simulink model "HPFilter"  (R2020b)
settings: Solver=VariableStepAuto  StartTime=0.0  StopTime=0.1  RelTol=1e-3
settings Model: Creator=Admin  LastModifiedBy=Admin

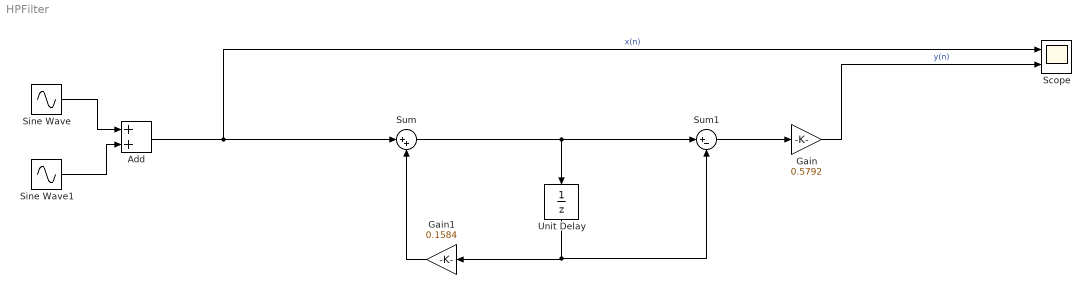
== system HPFilter ==
  Add : Sum
  Gain : Gain  Gain=0.5792
  Gain1 : Gain  Gain=0.1584
  Scope : Scope  NumInputPorts=2
  Sine Wave : Sin  Frequency=200/2*pi  SampleTime=0
  Sine Wave1 : Sin  Amplitude=0.25  Frequency=1000/2*pi  SampleTime=0
  Sum : Sum  Inputs=|++
  Sum1 : Sum  Inputs=|+-
  Unit Delay : UnitDelay  SampleTime=-1  HasFrameUpgradeWarning=on
  wires:
  Sum/1 -> Unit Delay/1, Sum1/1
  Sine Wave/1 -> Add/1
  Unit Delay/1 -> Sum1/2, Gain1/1
  Add/1 -> Scope/1, Sum/1  "x(n)"
  Sine Wave1/1 -> Add/2
  Gain/1 -> Scope/2  "y(n)"
  Sum1/1 -> Gain/1
  Gain1/1 -> Sum/2
